simulink model "abs_v12"  (R2020b)
settings: Solver=ode4  StartTime=0.0  StopTime=50  RelTol=1e-3
undefined symbols (not defined in the file or in its folder): A, c1, c2, c3, c4, Cd, d, F, H, jw, k, m, r, W
libraries: pid_lib x1
settings Model: Creator=K E S SRINIVAS  LastModifiedBy=K E S SRINIVAS
settings DataIOCC: ReturnWorkspaceOutputs=off

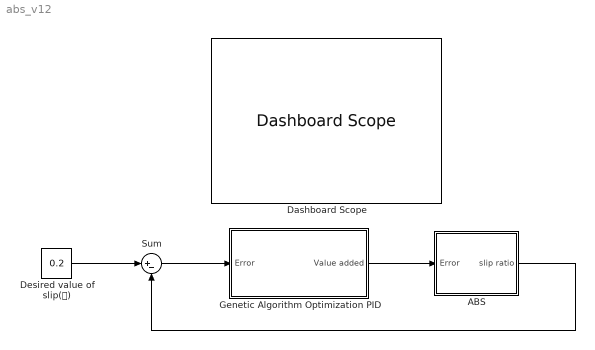
== system abs_v12 ==
  ABS : Subsystem
  Dashboard Scope : DashboardScope
  Desired value of slip(𝜆) : Constant  Value=0.2
  Genetic Algorithm Optimization PID : Subsystem
  Sum : Sum  Inputs=|+-
  wires:
  ABS/1(slip ratio) -> Sum/2
  Desired value of slip(𝜆)/1 -> Sum/1
  Genetic Algorithm Optimization PID/1(Value added) -> ABS/1(Error)
  Sum/1 -> Genetic Algorithm Optimization PID/1(Error)

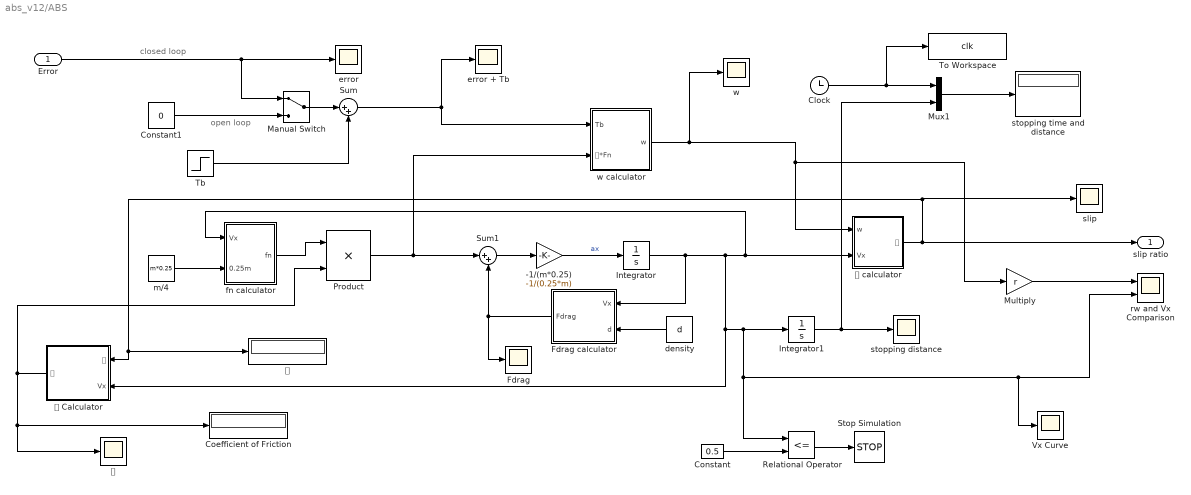
== system abs_v12/ABS ==
  note: closed loop
  note: open loop
  Error : Inport
  -1/(m*0.25) : Gain  Gain=-1/(0.25*m)
  Clock : Clock
  Coefficient of Friction : Display
  Constant : Constant  Value=0.5
  Constant1 : Constant  Value=0
  Fdrag : Scope
  Fdrag calculator : Subsystem
  Integrator : Integrator  InitialCondition=27.78  LimitOutput=on  LowerSaturationLimit=0
  Integrator1 : Integrator
  Manual Switch : ManualSwitch
  Multiply : Gain  Gain=r
  Mux1 : Mux  Inputs=2
  Product : Product
  Relational Operator : RelationalOperator  Operator=<=  OutDataTypeStr=boolean  RndMeth=Simplest
  Stop Simulation : Stop
  Sum : Sum  Inputs=|++
  Sum1 : Sum  Inputs=|++
  Tb : Step  Time=0  After=1200  SampleTime=0
  To Workspace : ToWorkspace  VariableName=clk  SaveFormat=Timeseries  SampleTime=-1
  Vx Curve : Scope
  density : Constant  Value=d
  error : Scope
  error + Tb : Scope
  fn calculator : Subsystem
  m/4 : Constant  Value=m*0.25
  "rw and Vx Comparison " : Scope  NumInputPorts=2
  slip : Scope
  stopping distance : Scope
  stopping time and distance : Display
  w : Scope
  w calculator : Subsystem
  𝜆 : Display
  𝜆 calculator : Subsystem
  𝜇 : Scope
  𝜇 Calculator : Subsystem
  slip ratio : Outport
  wires:
  𝜇 Calculator/1(𝜇) -> Product/2, 𝜇/1, Coefficient of Friction/1
  Integrator/1 -> "rw and Vx Comparison "/2, Vx Curve/1, Relational Operator/1, Integrator1/1, 𝜇 Calculator/2(Vx), 𝜆 calculator/2(Vx), fn calculator/1(Vx), Fdrag calculator/1(Vx)
  -1/(m*0.25)/1 -> Integrator/1  "ax"
  Relational Operator/1 -> Stop Simulation/1
  Constant/1 -> Relational Operator/2
  Sum/1 -> w calculator/1(Tb), error + Tb/1
  Error/1 -> Manual Switch/1, error/1
  Tb/1 -> Sum/2
  w calculator/1(w) -> Multiply/1, 𝜆 calculator/1(w), w/1
  𝜆 calculator/1(𝜆) -> slip/1, 𝜆/1, 𝜇 Calculator/1(𝜆), slip ratio/1
  Integrator1/1 -> Mux1/2, stopping distance/1
  Multiply/1 -> "rw and Vx Comparison "/1
  Clock/1 -> To Workspace/1, Mux1/1
  Mux1/1 -> stopping time and distance/1
  Constant1/1 -> Manual Switch/2
  Manual Switch/1 -> Sum/1
  Sum1/1 -> -1/(m*0.25)/1
  Fdrag calculator/1(Fdrag) -> Sum1/2, Fdrag/1
  Product/1 -> Sum1/1, w calculator/2(𝜇*Fn)
  fn calculator/1(fn) -> Product/1
  density/1 -> Fdrag calculator/2(d)
  m/4/1 -> fn calculator/2(0.25m)

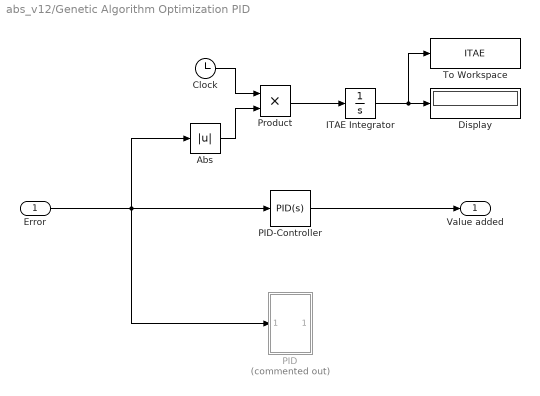
== system abs_v12/Genetic Algorithm Optimization PID ==
  Error : Inport
  Abs : Abs
  Clock : Clock
  Display : Display
  ITAE Integrator : Integrator
  PID : Subsystem  Commented=on
  PID-Controller : pid_lib/PID Controller  Controller=PID  Form=Parallel  TimeDomain=Continuous-time  UseExternalTs=off  SampleTime=-1  IntegratorMethod=Forward Euler  FilterMethod=Forward Euler  ControllerParametersSource=internal  P=90468  I=0  D=0  UseFilter=on  N=100  TunerSelectOption=Transfer Function Based (PID Tuner App)  InitialConditionSource=internal  InitialConditionForIntegrator=0  InitialConditionForFilter=0  DifferentiatorICPrevScaledInput=0  ExternalReset=none  TrackingMode=off  Kt=1  LimitOutput=off  SatLimitsSource=internal  UpperSaturationLimit=inf  LowerSaturationLimit=-inf  LinearizeAsGain=on  AntiWindupMode=none  Kb=1  POutMin=[]  POutMax=[]  IOutMin=[]  IOutMax=[]  DOutMin=[]  DOutMax=[]  NOutMin=[]  NOutMax=[]  SumOutMin=[]  SumOutMax=[]  SaturationOutMin=[]  SaturationOutMax=[]  PParamMin=[]  PParamMax=[]  IParamMin=[]  IParamMax=[]  DParamMin=[]  DParamMax=[]  NParamMin=[]  NParamMax=[]  KbParamMin=[]  KbParamMax=[]  KtParamMin=[]  KtParamMax=[]  KbOutMin=[]  KbOutMax=[]  KtOutMin=[]  KtOutMax=[]  IntegratorOutMin=[]  IntegratorOutMax=[]  FilterOutMin=[]  FilterOutMax=[]  SumI1OutMin=[]  SumI1OutMax=[]  SumI2OutMin=[]  SumI2OutMax=[]  SumI3OutMin=[]  SumI3OutMax=[]  SumI4OutMin=[]  SumI4OutMax=[]  SumDOutMin=[]  SumDOutMax=[]  DifferentiatorOutMin=[]  DifferentiatorOutMax=[]  FilterDiffOutCoefMin=[]  FilterDiffOutCoefMax=[]  ReciprocalOutMin=[]  ReciprocalOutMax=[]  SumDenOutMin=[]  SumDenOutMax=[]  SumNumOutMin=[]  SumNumOutMax=[]  DivideOutMin=[]  DivideOutMax=[]  UdiffTsProdOutMin=[]  UdiffTsProdOutMax=[]  NTsProdOutMin=[]  NTsProdOutMax=[]  UintegralTsProdOutMin=[]  UintegralTsProdOutMax=[]  UngainTsProdOutMin=[]  UngainTsProdOutMax=[]  IntegratorContinuousStateAttributes=''  IntegratorStateMustResolveToSignalObject=off  IntegratorRTWStateStorageClass=Auto  FilterContinuousStateAttributes=''  FilterStateMustResolveToSignalObject=off  FilterRTWStateStorageClass=Auto  ParallelPVariant=InternalParameters  IdealPVariant=Disabled  IVariant=InternalParameters  DVariant=InternalParameters  IntegratorVariant=Continuous  SatVariant=Disabled  AWVariant=Passthrough  PCopyVariant=Disabled  TRVariant=Disabled  FdbkBlocksVariant=Forward  IdealPFdbkVariant=Disabled  SatFdbkVariant=Disabled  DerivativeFilterVariant=ContFilter  NVariant=InternalParameters  NCopyVariant=Disabled  FilterICVariant=InternalICsFilter  IntegratorICVariant=InternalICs  ExternalResetVariant=Disabled  TRSumVariant=Passthrough  SumFdbkVariant=Disabled  SumVariant=Sum_PID  TsampFilterVariant=InternalTs  TsampNgainVariant=Passthrough  TsampIntegralVariant=Passthrough  ExternalSaturationOutDataTypeStr=Inherit: Same as second input
  Product : Product
  To Workspace : ToWorkspace  VariableName=ITAE  SampleTime=-1
  Value added : Outport
  wires:
  Error/1 -> PID-Controller/1, PID/1(In3), Abs/1
  Abs/1 -> Product/2
  Clock/1 -> Product/1
  ITAE Integrator/1 -> To Workspace/1, Display/1
  Product/1 -> ITAE Integrator/1
  PID-Controller/1 -> Value added/1

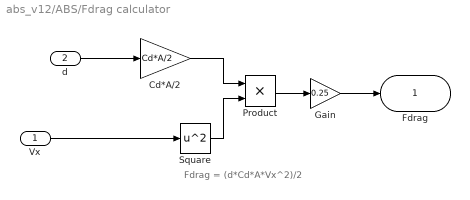
== system abs_v12/ABS/Fdrag calculator ==
  note: Fdrag = (d*Cd*A*Vx^2)/2
  Vx : Inport
  d : Inport  Port=2
  Cd*A/2 : Gain  Gain=Cd*A/2
  Gain : Gain  Gain=0.25
  Product : Product
  Square : Math  Operator=square  SaturateOnIntegerOverflow=on
  Fdrag : Outport
  wires:
  Square/1 -> Product/2
  d/1 -> Cd*A/2/1
  Cd*A/2/1 -> Product/1
  Product/1 -> Gain/1
  Vx/1 -> Square/1
  Gain/1 -> Fdrag/1

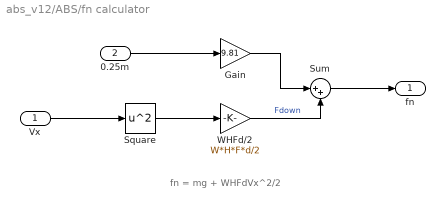
== system abs_v12/ABS/fn calculator ==
  note: fn = mg + WHFdVx^2/2
  Vx : Inport
  0.25m : Inport  Port=2
  Gain : Gain  Gain=9.81
  Square : Math  Operator=square  SaturateOnIntegerOverflow=on
  Sum : Sum  Inputs=|++
  WHFd/2 : Gain  Gain=W*H*F*d/2
  fn : Outport
  wires:
  Vx/1 -> Square/1
  Square/1 -> WHFd/2/1
  Sum/1 -> fn/1
  WHFd/2/1 -> Sum/2  "Fdown"
  0.25m/1 -> Gain/1
  Gain/1 -> Sum/1

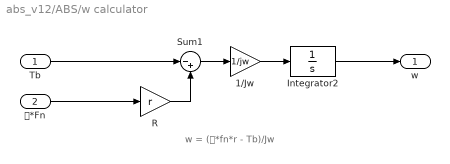
== system abs_v12/ABS/w calculator ==
  note: w = (𝜇*fn*r - Tb)/Jw
  Tb : Inport
  𝜇*Fn : Inport  Port=2
  1/Jw : Gain  Gain=1/jw
  Integrator2 : Integrator  InitialCondition=84.18  LimitOutput=on  UpperSaturationLimit=100000  LowerSaturationLimit=0.01  IgnoreLimit=on
  R : Gain  Gain=r
  Sum1 : Sum  Inputs=|-+
  w : Outport
  wires:
  Sum1/1 -> 1/Jw/1
  Tb/1 -> Sum1/1
  Integrator2/1 -> w/1
  𝜇*Fn/1 -> R/1
  1/Jw/1 -> Integrator2/1
  R/1 -> Sum1/2

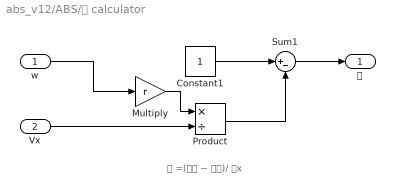
== system abs_v12/ABS/𝜆 calculator ==
  note: 𝜆 =(𝑉𝑥 − 𝜔𝑅)/ 𝑉x
  w : Inport
  Vx : Inport  Port=2
  Constant1 : Constant
  Multiply : Gain  Gain=r
  Product : Product  Inputs=*/
  Sum1 : Sum  Inputs=|+-
  𝜆 : Outport
  wires:
  w/1 -> Multiply/1
  Constant1/1 -> Sum1/1
  Vx/1 -> Product/2
  Multiply/1 -> Product/1
  Product/1 -> Sum1/2
  Sum1/1 -> 𝜆/1

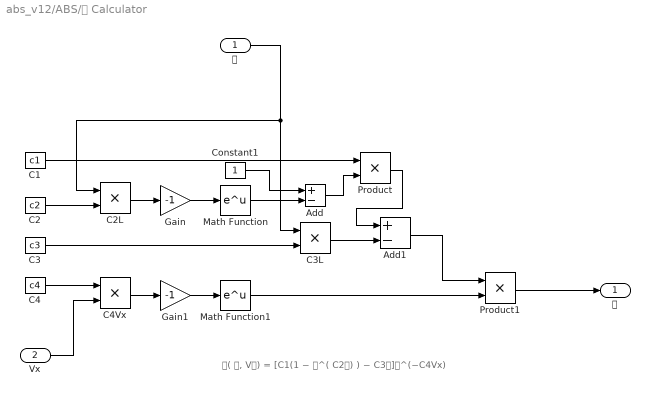
== system abs_v12/ABS/𝜇 Calculator ==
  note: 𝜇( 𝜆, V𝑥) = [C1(1 − 𝑒^( C2𝜆) ) − C3𝜆]𝑒^(−C4Vx)
  𝜆 : Inport
  Vx : Inport  Port=2
  Add : Sum  Inputs=+-
  Add1 : Sum  Inputs=+-
  C1 : Constant  Value=c1
  C2 : Constant  Value=c2
  C2L : Product
  C3 : Constant  Value=c3
  C3L : Product
  C4 : Constant  Value=c4
  C4Vx : Product
  Constant1 : Constant
  Gain : Gain  Gain=-1
  Gain1 : Gain  Gain=-1
  Math Function : Math  SaturateOnIntegerOverflow=on
  Math Function1 : Math  SaturateOnIntegerOverflow=on
  Product : Product
  Product1 : Product
  𝜇 : Outport
  wires:
  C2/1 -> C2L/2
  Gain/1 -> Math Function/1
  C1/1 -> Product/1
  C2L/1 -> Gain/1
  Constant1/1 -> Add/1
  Vx/1 -> C4Vx/2
  C4/1 -> C4Vx/1
  Add/1 -> Product/2
  Math Function/1 -> Add/2
  Gain1/1 -> Math Function1/1
  Math Function1/1 -> Product1/2
  C3L/1 -> Add1/2
  𝜆/1 -> C3L/1, C2L/1
  C4Vx/1 -> Gain1/1
  C3/1 -> C3L/2
  Product/1 -> Add1/1
  Add1/1 -> Product1/1
  Product1/1 -> 𝜇/1

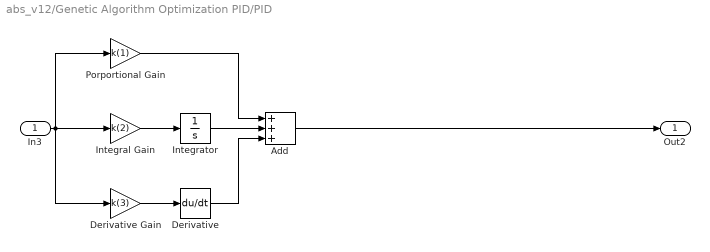
== system abs_v12/Genetic Algorithm Optimization PID/PID ==
  In3 : Inport
  Add : Sum  Inputs=+++
  Derivative : Derivative
  Derivative Gain : Gain  Gain=k(3)
  Integral Gain : Gain  Gain=k(2)
  Integrator : Integrator
  Porportional Gain : Gain  Gain=k(1)
  Out2 : Outport
  wires:
  Integral Gain/1 -> Integrator/1
  Porportional Gain/1 -> Add/1
  Derivative Gain/1 -> Derivative/1
  Derivative/1 -> Add/3
  Integrator/1 -> Add/2
  In3/1 -> Porportional Gain/1, Derivative Gain/1, Integral Gain/1
  Add/1 -> Out2/1
